simulink model "Lab_8_1"  (R2023a)
settings: Solver=VariableStepAuto  StartTime=0.0  StopTime=10.0  RelTol=1e-3
settings Model: Creator=mluser  LastModifiedBy=mluser

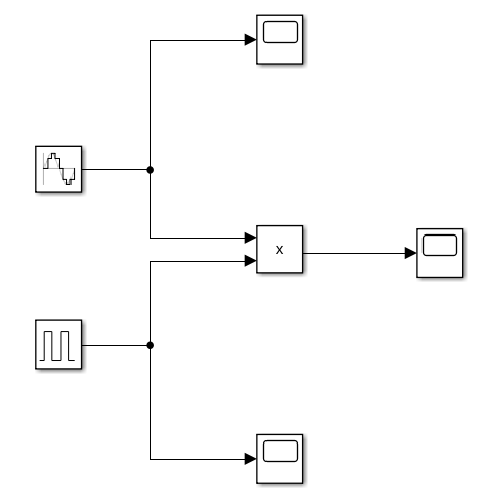
[thumbnail: Simulink's stored preview of the top-level diagram]
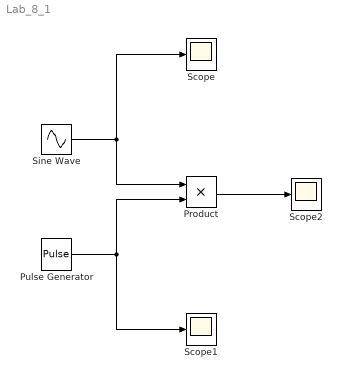
== system Lab_8_1 ==
  Product : Product
  Pulse Generator : DiscretePulseGenerator  PulseType=Time based  Period=0.8  PulseWidth=50
  Scope : Scope
  Scope1 : Scope
  Scope2 : Scope
  Sine Wave : Sin  SampleTime=0.01
  wires:
  Sine Wave/1 -> Product/1, Scope/1
  Product/1 -> Scope2/1
  Pulse Generator/1 -> Product/2, Scope1/1
